simulink model "quad_new_leg_simple_strategy"  (R2018a)
settings: Solver=ode15s  StartTime=0.0  StopTime=10.0  RelTol=1e-3
values from neighbouring files (symbols this model uses):
  X = ([-L/2, L/2, L/2, -L/2])    [draw_cube.m]
  Y = ([-W/2, -W/2, W/2, W/2])    [draw_cube.m]
undefined symbols (not defined in the file or in its folder): body, ctrl, ground, planner, Z
libraries: nesl_utility x71, sm_lib x41, simulink x29, Contact_Forces_Lib x4, Parts_Lib x4, sharedtransform x1
(part 4 of 4)

== matlab function quad_new_leg_simple_strategy/QuadCtrl ==
  data: fl_ang input; tgt_ctrl_fl output; fr_ang input; rl_ang input; rr_ang input; contact_state input; body_R input; sensing_info input; tgt_ctrl_fr output; tgt_ctrl_rl output; tgt_ctrl_rr output; t input; body parameter; planner parameter; debug output
function [tgt_ctrl_fl,tgt_ctrl_fr,tgt_ctrl_rl,tgt_ctrl_rr, debug] = controller(fl_ang, fr_ang, rl_ang, rr_ang, contact_state, body_R, sensing_info, t, body, planner)

fl_ang_s = fl_ang(1); fl_ang_u = fl_ang(2); fl_ang_k = fl_ang(3);
fr_ang_s = fr_ang(1); fr_ang_u = fr_ang(2); fr_ang_k = fr_ang(3);
rl_ang_s = rl_ang(1); rl_ang_u = rl_ang(2); rl_ang_k = rl_ang(3);
rr_ang_s = rr_ang(1); rr_ang_u = rr_ang(2); rr_ang_k = rr_ang(3);
% forward kinematics
fl_end_effector = forward_kinematics(fl_ang_s, fl_ang_u, fl_ang_k, body); 
rl_end_effector = forward_kinematics(rl_ang_s, rl_ang_u, rl_ang_k, body);
fr_end_effector = forward_kinematics(fr_ang_s, fr_ang_u, fr_ang_k, body);
rr_end_effector = forward_kinematics(rr_ang_s, rr_ang_u, rr_ang_k, body); 

% distance from center of mass to shoulder
fl_offset = [body.shoulder_distance;body.y_length/2+body.shoulder_size/2;0];
fr_offset = [body.shoulder_distance;-body.y_length/2-body.shoulder_size/2;0];
rl_offset = [-body.shoulder_distance;body.y_length/2+body.shoulder_size/2;0];
rr_offset = [-body.shoulder_distance;-body.y_length/2-body.shoulder_size/2;0];

%virtual leg1
virtual_leg1 = (fl_end_effector + fl_offset + rr_end_effector + rr_offset)*0.5;
%virtual leg2
virtual_leg2 = (fr_end_effector + fr_offset + rl_end_effector + rl_offset)*0.5;

circle_percent = t/planner.time_circle;
     
normal_virtual_leg1 = [0;0;planner.stand_height];
normal_virtual_leg2 = [0;0;planner.stand_height];
delta_ang = planner.swing_ang;
move_theta1 = delta_ang*sin(2*pi/planner.time_circle*t);

debug = move_theta1;
move_leg_y = [cos(move_theta1) 0 sin(move_theta1);
                            0 1               0;
             -sin(move_theta1) 0 cos(move_theta1)];
tgt_virtual_leg1 = move_leg_y*normal_virtual_leg1;

tgt_virtual_leg2 = move_leg_y'*normal_virtual_leg2;
         
has_u_ctrl = [1 1 1 1];

move_fl_end_effector = body_R*tgt_virtual_leg1;
move_rr_end_effector = body_R*tgt_virtual_leg1;
move_fr_end_effector = body_R*tgt_virtual_leg2;
move_rl_end_effector = body_R*tgt_virtual_leg2;

%% fl to joint
[inv_s,inv_u,inv_k] = inverse_kinematics(move_fl_end_effector, body);
fl_tgt_ang_s = inv_s; 
fl_tgt_ang_u = inv_u;       
fl_tgt_ang_k = inv_k; 
tgt_ctrl_fl = [fl_tgt_ang_s;fl_tgt_ang_u;fl_tgt_ang_k;has_u_ctrl(1)];

%% fr to joint
[inv_s,inv_u,inv_k] = inverse_kinematics(move_fr_end_effector, body);
fr_tgt_ang_s = inv_s;
fr_tgt_ang_u = inv_u;
fr_tgt_ang_k = inv_k;
tgt_ctrl_fr = [fr_tgt_ang_s;fr_tgt_ang_u;fr_tgt_ang_k;has_u_ctrl(2)];

%% rl to joint
[inv_s,inv_u,inv_k] = inverse_kinematics(move_rl_end_effector, body);
rl_tgt_ang_s = inv_s;
rl_tgt_ang_u = inv_u;
rl_tgt_ang_k = inv_k;
tgt_ctrl_rl = [rl_tgt_ang_s;rl_tgt_ang_u;rl_tgt_ang_k;has_u_ctrl(3)];

%% rr to joint
[inv_s,inv_u,inv_k] = inverse_kinematics(move_rr_end_effector, body);
rr_tgt_ang_s = inv_s;
rr_tgt_ang_u = inv_u;
rr_tgt_ang_k = inv_k; 
tgt_ctrl_rr = [rr_tgt_ang_s;rr_tgt_ang_u;rr_tgt_ang_k;has_u_ctrl(4)];
